simulink model "BLDCmotorControl_FOC_R2017b_fixdt"  (R2017b)
settings: Solver=FixedStepDiscrete  StartTime=0  StopTime=0.5  FixedStep=Ts  MaxStep=1e-6  RelTol=1e-6  AbsTol=1e-6  EnableMultiTasking=on
PreLoadFcn:
  | addpath(pwd);
  | addpath(genpath('01_Libraries'));
  | addpath(genpath('02_Figures'));
  | addpath(genpath('03_CreateParamTable'));
InitFcn:
  | init_model;
values from neighbouring files (symbols this model uses):
  a_elecAngle = 60    [init_model.m]
  a_elecPeriod = 360    [init_model.m]
  a_phaAdvMax = 25    [init_model.m]
  b_diagEna = 1    [init_model.m]
  b_fieldWeakEna = 0    [init_model.m]
  cf_currFilt = 0.12    [init_model.m]
  cf_idKi = 60 / (f_ctrl/3)    (= 0.01125)    [init_model.m]
  cf_idKp = 0.2    [init_model.m]
  cf_iqKi = 100 / (f_ctrl/3)    (= 0.01875)    [init_model.m]
  cf_iqKiLimProt = 60 / (f_ctrl/3)    (= 0.01125)    [init_model.m]
  cf_iqKp = 0.3    [init_model.m]
  cf_KbLimProt = 1000 / (f_ctrl/3)    (= 0.1875)    [init_model.m]
  cf_nKi = 20.4 / (f_ctrl/3)    (= 0.003825)    [init_model.m]
  cf_nKiLimProt = 20 / (f_ctrl/3)    (= 0.00375)    [init_model.m]
  cf_nKp = 1.18    [init_model.m]
  cf_speedCoef = round(f_ctrl * a_mechAngle * (pi/180) * (30/pi))    [init_model.m]
  CTRL_COM = 0    [init_model.m]
  CTRL_FOC = 2    [init_model.m]
  CTRL_SIN = 1    [init_model.m]
  dV_openRate = 1000 / (f_ctrl/3)    (= 0.1875)    [init_model.m]
  dz_cntTrnsDetHi = 40    [init_model.m]
  dz_cntTrnsDetLo = 20    [init_model.m]
  i_max = i_max * i_sca    (= 750)    [init_model.m]
  id_fieldWeakMax = 5 * i_sca    (= 250)    [init_model.m]
  iq_maxSca_M1 = sqrt(1 - iq_maxSca_XA.^2)    [init_model.m]
  n_commAcvLo = 15    [init_model.m]
  n_commDeacvHi = 30    [init_model.m]
  n_fieldWeakAuthHi = 400    [init_model.m]
  n_fieldWeakAuthLo = 300    [init_model.m]
  n_max = 1000    [init_model.m]
  n_polePairs = 15    [init_model.m]
  n_stdStillDet = 3    [init_model.m]
  OPEN_MODE = 0    [init_model.m]
  r_cos_M1 = cos((a_elecAngle_XA + 0)*(pi/180))    [init_model.m]
  r_errInpTgtThres = 600    [init_model.m]
  r_fieldWeakHi = 1500    [init_model.m]
  r_fieldWeakLo = 1000    [init_model.m]
  r_sin3PhaA_M1 = sin3Arm + A*r_sinPhaA_M1    [init_model.m]
  r_sin3PhaB_M1 = sin3Arm + A*r_sinPhaB_M1    [init_model.m]
  r_sin3PhaC_M1 = sin3Arm + A*r_sinPhaC_M1    [init_model.m]
  r_sin_M1 = sin((a_elecAngle_XA + 0)*(pi/180))    [init_model.m]
  SPD_MODE = 2    [init_model.m]
  t_errDequal = 1.80 * f_ctrl/3    (= 9600)    [init_model.m]
  t_errQual = 0.24 * f_ctrl/3    (= 1280)    [init_model.m]
  TRQ_MODE = 3    [init_model.m]
  Ts = 5e-6    (= 5e-06)    [init_model.m]
  Ts_ctrl = 6e-5    (= 6e-05)    [init_model.m]
  Vd_max = 1000 - V_margin    (= 900)    [init_model.m]
  vec_hallToPos = [0 2 0 1 4 3 5 0]    [init_model.m]
  VLT_MODE = 1    [init_model.m]
  Vq_max_M1 = sqrt(Vd_max^2 - Vq_max_XA.^2)    [init_model.m]
  z_commutMap_M1 = [-1 -1  0  1  1  0 ... (first row only)    [init_model.m]
  z_ctrlModReq = VLT_MODE    (= 1)    [init_model.m]
  z_ctrlTypSel = 2    [init_model.m]
  z_maxCntRst = 2000    [init_model.m]
  z_selPhaCurMeasABC = 0    [init_model.m]
undefined symbols (not defined in the file or in its folder): DiscIntNeverNeededParam, sigbuilder_block
libraries: BLDC_controller_Lib x15, simulink x14, powerlib x6, pePwmGenerator x1
(part 1 of 4)
Description:
  | This model implements FOC controller for a BLDC motor.
  | The controller is capable for embedded code generation.
  | 
  | Copyright © Emanuel FERU
settings Model: ExtModeAutoUpdateStatusClock=off  TunableVars=Vd_max,Vq_max_M1,Vq_max_XA,a_phaAdvMax,b_diagEna,b_fieldWeakEna,b_selPhaABCurrMeas,cf_KbLimProt,cf_currFilt,cf_idKi,cf_idKp,cf_iqKi,cf_iqKiLimProt,cf_iqKp,cf_nKi,cf_nKiLimProt,cf_nKp,cf_speedCoef,dV_openRate,dz_cntTrnsDetHi,dz_cntTrnsDetLo,i_max,id_fieldWeakMax,n_commAcvLo,n_commDeacvHi,n_fieldWeakAuthHi,n_fieldWeakAuthLo,n_max,n_stdStillDet,r_errInpTgtThres,r_fieldWeakHi,r_fieldWeakLo,t_errDequal,t_errQual,z_ctrlTypSel,z_maxCntRst,z_selPhaCurMeasABC  TunableVarsStorageClass=Auto,Auto,Auto,Auto,Auto,Auto,Auto,Auto,Auto,Auto,Auto,Auto,Auto,Auto,Auto,Auto,Auto,Auto,Auto,Auto,Auto,Auto,Auto,Auto,Auto,Auto,Auto,Auto,Auto,Auto,Auto,Auto,Auto,Auto,Auto,Auto,Auto  TunableVarsTypeQualifier=,,,,,,,,,,,,,,,,,,,,,,,,,,,,,,,,,,,,  Creator=MathWorks  LastModifiedBy=eferu
settings SolverCC: AutoInsertRateTranBlk=on
settings DataIOCC: LimitDataPoints=on  SaveFormat=Array  ReturnWorkspaceOutputs=on  SignalLoggingName=sigsOut
settings OptimizationCC: DefaultParameterBehavior=Inlined  UseDivisionForNetSlopeComputation=on  UseFloatMulNetSlope=on  UseSpecifiedMinMax=on  InlineInvariantSignals=on  PassReuseOutputArgsAs=Individual arguments  ExpressionDepthLimit=2147483647  ZeroExternalMemoryAtStartup=off  ZeroInternalMemoryAtStartup=off  NoFixptDivByZeroProtection=on  EfficientFloat2IntCast=on  LifeSpan=1  OptimizeBlockOrder=speed  DifferentSizesBufferReuse=on
settings DebuggingCC: ReadBeforeWriteMsg=DisableAll  WriteAfterWriteMsg=DisableAll  WriteAfterReadMsg=DisableAll  UnderspecifiedInitializationDetection=Classic  InheritedTsInSrcMsg=none  MultiTaskDSMMsg=none  MultiTaskCondExecSysMsg=none  ParameterTunabilityLossMsg=error  FcnCallInpInsideContextMsg=warning  UnconnectedInputMsg=error  UnconnectedOutputMsg=error  UnconnectedLineMsg=error  StateNameClashWarn=warning  SFUnexpectedBacktrackingDiag=warning  SFNoUnconditionalDefaultTransitionDiag=warning  SFExecutionAtInitializationDiag=none
settings HardwareCC: ProdBitPerPointer=32  ProdBitPerSizeT=32  ProdBitPerPtrDiffT=32  ProdLargestAtomicInteger=Long  ProdLargestAtomicFloat=Double  ProdWordSize=32  ProdHWDeviceType=ARM Compatible->ARM Cortex  TargetBitPerPointer=64  TargetBitPerSizeT=64  TargetBitPerPtrDiffT=64  TargetLongLongMode=on  TargetIntDivRoundTo=Zero  TargetEndianess=LittleEndian  TargetWordSize=64  TargetHWDeviceType=MATLAB Host  ProdEqTarget=off
settings ModelReferenceCC: UpdateModelReferenceTargets=IfOutOfDate  PropagateSignalLabelsOutOfModel=off
settings SFSimCC: SFSimEcho=off  MATLABDynamicMemAlloc=off
settings RTWCC: SystemTargetFile=ert.tlc  GenCodeOnly=on  TemplateMakefile=ert_default_tmf  GenerateReport=on  BuildConfiguration=Faster Runs  IncludeHyperlinkInReport=on  LaunchReport=on  GenerateTraceInfo=on  GenerateTraceReport=on  GenerateTraceReportSl=on  GenerateTraceReportSf=on  GenerateTraceReportEml=on  GenerateWebview=on  GenerateCodeMetricsReport=on  GenerateCodeReplacementReport=on
settings CodeAppCC: ForceParamTrailComments=on  IgnoreCustomStorageClasses=off  OperatorAnnotations=on  SimulinkDataObjDesc=on  SFDataObjDesc=on  CustomSymbolStrGlobalVar=rt$N$M  CustomSymbolStrType=$N$M  CustomSymbolStrFcn=$N$M$F  CustomSymbolStrMacro=$N$M  InsertBlockDesc=on
settings ERTTargetCC: GenerateSampleERTMain=on  IncludeMdlTerminateFcn=off  CombineSignalStateStructs=on  SuppressErrorStatus=on  MultiInstanceERTCode=on  CodeInterfacePackaging=Reusable function  SupportNonFinite=off  SupportComplex=off  InlinedParameterPlacement=NonHierarchical  RootIOFormat=Part of model data structure  ERTCustomFileTemplate=example_file_process.tlc  ERTFilePackagingFormat=CompactWithDataFile  PreserveStaticInFcnDecls=off
settings ConfigComp: CovMetricSettings=dw  CovHtmlReporting=on  CovSaveCumulativeToWorkspaceVar=on  CovSaveSingleToWorkspaceVar=on  CovExternalEMLEnable=off  CovSFcnEnable=off
settings SimscapeCC: SimscapeNormalizeSystem=off

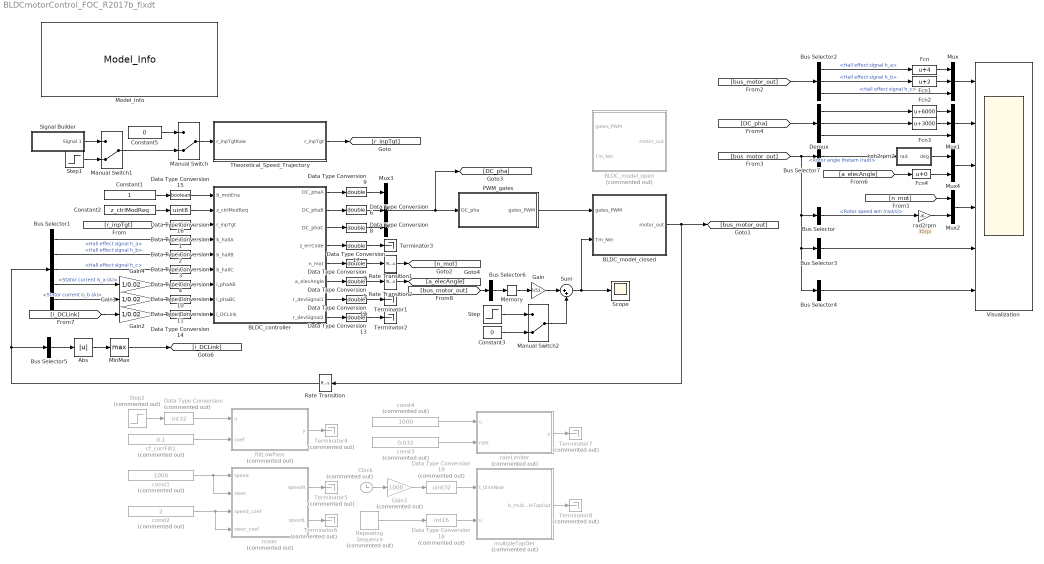
== system BLDCmotorControl_FOC_R2017b_fixdt ==
  Abs : Abs
  BLDC_controller : Subsystem  TreatAsAtomicUnit=on  SystemSampleTime=Ts_ctrl
  BLDC_model_closed : Subsystem
      mask help: Simulink:masks:GenSFuncDesc_MD
      mask Help: eval('feval(''rtwprivate'',''rtwhelpview'',''rtw_sfcn_block'')');
  BLDC_model_open : Subsystem  Commented=on
  Bus Selector : BusSelector  OutputSignals=Rotor speed wm (rad/s)
  Bus Selector1 : BusSelector  OutputSignals=Hall effect signal h_a,Hall effect signal h_b,Hall effect signal h_c,Stator current is_a (A),Stator current is_b (A)
  Bus Selector2 : BusSelector  OutputSignals=Hall effect signal h_a,Hall effect signal h_b,Hall effect signal h_c
  Bus Selector3 : BusSelector  OutputSignals=Stator current is_a (A),Stator current is_b (A),Stator current is_c (A),Electromagnetic torque Te (N*m)  OutputAsBus=on
  Bus Selector4 : BusSelector  OutputSignals=Stator back EMF e_a (V),Stator back EMF e_b (V),Stator back EMF e_cV)  OutputAsBus=on
  Bus Selector5 : BusSelector  OutputSignals=Stator current is_a (A),Stator current is_b (A),Stator current is_c (A)  OutputAsBus=on
  Bus Selector6 : BusSelector  OutputSignals=Rotor speed wm (rad/s)  OutputAsBus=on
  Bus Selector7 : BusSelector  OutputSignals=Rotor angle thetam (rad)
  Clock : Clock  Commented=on
  Constant1 : Constant  OutDataTypeStr=double
  Constant2 : Constant  Value=z_ctrlModReq  OutDataTypeStr=double
  Constant3 : Constant  Value=0  OutDataTypeStr=double
  Constant5 : Constant  Value=0  OutDataTypeStr=double
  Data Type Conversion : DataTypeConversion  Commented=on  OutDataTypeStr=int32
  Data Type Conversion{1,10..11,14} (4 alike) : DataTypeConversion  OutDataTypeStr=int16  RndMeth=Zero
  Data Type Conversion{5..9,12..13,17} (8 alike) : DataTypeConversion  OutDataTypeStr=double  RndMeth=Zero
  Data Type Conversion15 : DataTypeConversion  OutDataTypeStr=boolean  RndMeth=Zero
  Data Type Conversion{2..4,16} (4 alike) : DataTypeConversion  OutDataTypeStr=uint8  RndMeth=Zero
  Data Type Conversion18 : DataTypeConversion  Commented=on  OutDataTypeStr=int16
  Data Type Conversion19 : DataTypeConversion  Commented=on  OutDataTypeStr=uint32
  Demux : Demux  Outputs=3
  Fcn : Fcn  Expr=u+4
  Fcn1 : Fcn  Expr=u+2
  Fcn2 : Fcn  Expr=u+6000
  Fcn3 : Fcn  Expr=u+3000
  Fcn4 : Fcn  Expr=u+0
  Gain : Gain  Gain=5/52
  Gain1 : Gain  Tag=struct('comment',struct('text','','placement',1),'logdata',struct('maxnumvals',inf,'plotchannels',[],'loggingmode',3,'channels',1),'output',struct('variable','','description','','name','$S_$B','width',1,'address','','max',NaN,'min',NaN,'class','default','type','CONTINUOUS','scaling','','lsb',1,'offset',0,'arb',0,'freeze',1,'unit','','autoscalingmode',1,'lowerheadroom',1,'upperheadroom',1,'headroomunit','bit','keepdatatype',1,'checkmin',0,'checkmax',0,'castoutput',0,'show',0),'gain',struct('variable','','description','','name','$S_$B_gain','width',1,'address','','max',NaN,'min',NaN,'class','default','type','CONTINUOUS','scaling','','lsb',1,'offset',0,'arb',0,'freeze',1,'unit','','keepdatatype',1,'value','1','scalar',0,'tolerance',1),'scalingvalid',0,'date',730486)  Gain=1/0.02  RndMeth=Zero  SaturateOnIntegerOverflow=on  OutDataTypeStr=Inherit: Same as input  ParamDataTypeStr=Inherit: Same as input
  Gain2 : Gain  Tag=struct('comment',struct('text','','placement',1),'logdata',struct('maxnumvals',inf,'plotchannels',[],'loggingmode',3,'channels',1),'output',struct('variable','','description','','name','$S_$B','width',1,'address','','max',NaN,'min',NaN,'class','default','type','CONTINUOUS','scaling','','lsb',1,'offset',0,'arb',0,'freeze',1,'unit','','autoscalingmode',1,'lowerheadroom',1,'upperheadroom',1,'headroomunit','bit','keepdatatype',1,'checkmin',0,'checkmax',0,'castoutput',0,'show',0),'gain',struct('variable','','description','','name','$S_$B_gain','width',1,'address','','max',NaN,'min',NaN,'class','default','type','CONTINUOUS','scaling','','lsb',1,'offset',0,'arb',0,'freeze',1,'unit','','keepdatatype',1,'value','1','scalar',0,'tolerance',1),'scalingvalid',0,'date',730486)  Gain=1/0.02  RndMeth=Zero  SaturateOnIntegerOverflow=on  OutDataTypeStr=Inherit: Same as input  ParamDataTypeStr=Inherit: Same as input
  Gain3 : Gain  Tag=struct('comment',struct('text','','placement',1),'logdata',struct('maxnumvals',inf,'plotchannels',[],'loggingmode',3,'channels',1),'output',struct('variable','','description','','name','$S_$B','width',1,'address','','max',NaN,'min',NaN,'class','default','type','CONTINUOUS','scaling','','lsb',1,'offset',0,'arb',0,'freeze',1,'unit','','autoscalingmode',1,'lowerheadroom',1,'upperheadroom',1,'headroomunit','bit','keepdatatype',1,'checkmin',0,'checkmax',0,'castoutput',0,'show',0),'gain',struct('variable','','description','','name','$S_$B_gain','width',1,'address','','max',NaN,'min',NaN,'class','default','type','CONTINUOUS','scaling','','lsb',1,'offset',0,'arb',0,'freeze',1,'unit','','keepdatatype',1,'value','1','scalar',0,'tolerance',1),'scalingvalid',0,'date',730486)  Commented=on  Gain=1000  RndMeth=Zero  SaturateOnIntegerOverflow=on  OutDataTypeStr=Inherit: Same as input  ParamDataTypeStr=Inherit: Same as input
  Gain4 : Gain  Tag=struct('comment',struct('text','','placement',1),'logdata',struct('maxnumvals',inf,'plotchannels',[],'loggingmode',3,'channels',1),'output',struct('variable','','description','','name','$S_$B','width',1,'address','','max',NaN,'min',NaN,'class','default','type','CONTINUOUS','scaling','','lsb',1,'offset',0,'arb',0,'freeze',1,'unit','','autoscalingmode',1,'lowerheadroom',1,'upperheadroom',1,'headroomunit','bit','keepdatatype',1,'checkmin',0,'checkmax',0,'castoutput',0,'show',0),'gain',struct('variable','','description','','name','$S_$B_gain','width',1,'address','','max',NaN,'min',NaN,'class','default','type','CONTINUOUS','scaling','','lsb',1,'offset',0,'arb',0,'freeze',1,'unit','','keepdatatype',1,'value','1','scalar',0,'tolerance',1),'scalingvalid',0,'date',730486)  Gain=1/0.02  RndMeth=Zero  SaturateOnIntegerOverflow=on  OutDataTypeStr=Inherit: Same as input  ParamDataTypeStr=Inherit: Same as input
  Manual Switch : ManualSwitch  CurrentSetting=0
  Manual Switch1 : ManualSwitch  CurrentSetting=0
  Manual Switch2 : ManualSwitch  CurrentSetting=0
  Memory : Memory
  MinMax : MinMax  Function=max
  Model_Info : BLDC_controller_Lib/Model_Info
  Mux : Mux  Inputs=3
  Mux1 : Mux  Inputs=3
  Mux2 : Mux  Inputs=2
  Mux3 : Mux  Inputs=3
  Mux4 : Mux  Inputs=2
  PWM_gates : Subsystem
  Rate Transition : RateTransition  Integrity=off  Deterministic=off
  Rate Transition1 : RateTransition
  Rate Transition2 : RateTransition
  Repeating Sequence : simulink/Sources/Repeating Sequence  Commented=on  rep_seq_t=[0 0.4 0.8 1.2 1.6 3]  rep_seq_y="[0 900  0  900 0 0]"
  Scope : Scope
  Signal Builder : Subsystem  Tag=STV Subsys  LoadFcn=sigbuilder_block('load');  StartFcn=sigbuilder_block('start');  StopFcn=sigbuilder_block('stop');  ClipboardFcn=sigbuilder_block('clipboard');  mask(Sigbuilder block){tuvar=[0:10]}
      mask help: Simulink:masks:SigbuilderBlock_MD
      mask init:
      | if ~strcmp(get_param(bdroot(gcbh),'SimulationStatus'),'stopped') tuvar = sigbuilder_block('maskInit'); end
      settings: CopyFcn=sigbuilder_block('copy');  DeleteFcn=sigbuilder_block('delete');  ModelCloseFcn=sigbuilder_block('modelClose');  PreSaveFcn=sigbuilder_block('preSave');  PauseFcn=sigbuilder_block('pause');  ContinueFcn=sigbuilder_block('continue');  NameChangeFcn=sigbuilder_block('namechange');  OpenFcn=sigbuilder_block('open',[141.283 165.057 550.868 400.075 ]);  CloseFcn=sigbuilder_block('close');
      mask Display: plot(0, 0, 100, 100,[2, 2, 32, 32, 2], [68, 8, 8, 68, 68],[32, 2], [38, 38], [32, 19, 2],[53, 60, 44], [32, 17, 17, 2],[16, 16, 31, 31]);txt = getActiveGroup(gcbh);text(2, 100, txt,'verticalAlignment', 'top');
  Step : Step  Time=0.25  Before=-5  After=5  SampleTime=0
  Step1 : Step  Time=0.25  Before=1500  After=-1500
  Step2 : Step  Commented=on  Time=0.25  Before=20000  After=0  SampleTime=0
  Sum : Sum  Inputs=|++
  Terminator1 : Terminator
      settings: Tag=Controls_Lib  Description=Terminator  CopyFcn=Lib_CopyFcn(gcb);  PreDeleteFcn=Lib_PreDeleteFcn(gcb);
  Terminator2 : Terminator
      settings: Tag=Controls_Lib  Description=Terminator  CopyFcn=Lib_CopyFcn(gcb);  PreDeleteFcn=Lib_PreDeleteFcn(gcb);
  Terminator3 : Terminator
      settings: Tag=Controls_Lib  Description=Terminator  CopyFcn=Lib_CopyFcn(gcb);  PreDeleteFcn=Lib_PreDeleteFcn(gcb);
  Terminator{4..8} (5 alike) : Terminator  Commented=on
      settings: Tag=Controls_Lib  Description=Terminator  CopyFcn=Lib_CopyFcn(gcb);  PreDeleteFcn=Lib_PreDeleteFcn(gcb);
  Theoretical_Speed_Trajectory : Subsystem
  Visualization : Scope  NumInputPorts=6
  cf_currFilt1 : Constant  Commented=on  Value=0.1  OutDataTypeStr=fixdt(0,16,16)
  const1 : Constant  Commented=on  Value=1000  OutDataTypeStr=fixdt(1,16,4)
  const2 : Constant  Commented=on  Value=2  OutDataTypeStr=fixdt(1,16,14)
  const3 : Constant  Commented=on  Value=0.032  OutDataTypeStr=fixdt(1,16,4)
  const4 : Constant  Commented=on  Value=1000  OutDataTypeStr=int16
  filtLowPass : Subsystem  Commented=on  TreatAsAtomicUnit=on  SystemSampleTime=Ts_ctrl
      settings: RTWFcnNameOpts=Use subsystem name
  kph2rpm2 : Subsystem
  mixer : Subsystem  Commented=on  TreatAsAtomicUnit=on  SystemSampleTime=Ts_ctrl
      settings: RTWFcnNameOpts=Use subsystem name
  multipleTapDet : Subsystem  Commented=on  TreatAsAtomicUnit=on
      settings: RTWFcnNameOpts=Use subsystem name
  rad2rpm : Gain  Gain=30/pi
  rateLimiter : Subsystem  Commented=on  TreatAsAtomicUnit=on  SystemSampleTime=Ts_ctrl
      settings: RTWFcnNameOpts=Use subsystem name
  wires:
  Mux2/1 -> Visualization/4
  Bus Selector/1 -> rad2rpm/1  "<Rotor speed wm (rad/s)>"
  Bus Selector2/3 -> Mux/3  "<Hall effect signal h_c>"
  Bus Selector2/2 -> Fcn1/1  "<Hall effect signal h_b>"
  Bus Selector2/1 -> Fcn/1  "<Hall effect signal h_a>"
  Fcn1/1 -> Mux/2
  Mux/1 -> Visualization/1
  Fcn/1 -> Mux/1
  Demux/1 -> Fcn2/1
  Demux/2 -> Fcn3/1
  Fcn2/1 -> Mux1/1
  Fcn3/1 -> Mux1/2
  Demux/3 -> Mux1/3
  Mux1/1 -> Visualization/2
  Bus Selector4/1 -> Visualization/6
  rad2rpm/1 -> Mux2/2
  BLDC_controller/5(n_mot) -> Data Type Conversion7/1
  Sum/1 -> BLDC_model_closed/2(Tm_Nm), Scope/1
  Bus Selector1/2 -> Data Type Conversion3/1  "<Hall effect signal h_b>"
  Bus Selector1/1 -> Data Type Conversion2/1  "<Hall effect signal h_a>"
  Bus Selector1/3 -> Data Type Conversion4/1  "<Hall effect signal h_c>"
  Data Type Conversion2/1 -> BLDC_controller/4("b_hallA ")
  Data Type Conversion3/1 -> BLDC_controller/5(b_hallB)
  Data Type Conversion4/1 -> BLDC_controller/6(b_hallC)
  Theoretical_Speed_Trajectory/1(r_inpTgt) -> [r_inpTgt]
  [r_inpTgt] -> Data Type Conversion1/1
  Data Type Conversion1/1 -> BLDC_controller/3(r_inpTgt)
  BLDC_controller/2(DC_phaB) -> Data Type Conversion6/1
  BLDC_controller/3(DC_phaC) -> Data Type Conversion8/1
  BLDC_controller/1(DC_phaA) -> Data Type Conversion9/1
  BLDC_controller/6(a_elecAngle) -> Data Type Conversion5/1
  Mux3/1 -> [DC_pha], PWM_gates/1(DC_pha)
  PWM_gates/1(gates_PWM) -> BLDC_model_closed/1(gates_PWM)
  Data Type Conversion7/1 -> Rate Transition1/1
  [n_mot] -> Mux2/1
  [bus_motor_out] -> Bus Selector2/1
  [bus_motor_out] -> Bus Selector7/1, Bus Selector3/1, Bus Selector4/1, Bus Selector/1
  [DC_pha] -> Demux/1
  Manual Switch/1 -> Theoretical_Speed_Trajectory/1(r_inpTgtRaw)
  Constant5/1 -> Manual Switch/1
  Signal Builder/1(Signal 1) -> Manual Switch1/1
  Manual Switch1/1 -> Manual Switch/2
  Step1/1 -> Manual Switch1/2
  Data Type Conversion5/1 -> Rate Transition2/1
  Data Type Conversion8/1 -> Mux3/3
  Data Type Conversion6/1 -> Mux3/2
  Data Type Conversion9/1 -> Mux3/1
  Data Type Conversion10/1 -> BLDC_controller/7(i_phaAB)
  Data Type Conversion11/1 -> BLDC_controller/8(i_phaBC)
  Gain4/1 -> Data Type Conversion10/1
  Gain1/1 -> Data Type Conversion11/1
  BLDC_controller/7(r_devSignal1) -> Data Type Conversion12/1
  Data Type Conversion13/1 -> Terminator2/1
  BLDC_controller/8(r_devSignal2) -> Data Type Conversion13/1
  Gain2/1 -> Data Type Conversion14/1
  Data Type Conversion14/1 -> BLDC_controller/9(i_DCLink)
  [i_DCLink] -> Gain2/1
  Bus Selector1/4 -> Gain4/1  "<Stator current is_a (A)>"
  Bus Selector1/5 -> Gain1/1  "<Stator current is_b (A)>"
  Data Type Conversion15/1 -> BLDC_controller/1(b_motEna)
  Constant1/1 -> Data Type Conversion15/1
  [bus_motor_out] -> Bus Selector6/1
  Bus Selector6/1 -> Memory/1
  Gain/1 -> Sum/1
  Data Type Conversion16/1 -> BLDC_controller/2(z_ctrlModReq)
  Constant2/1 -> Data Type Conversion16/1
  Rate Transition/1 -> Bus Selector1/1, Bus Selector5/1
  Memory/1 -> Gain/1
  Step/1 -> Manual Switch2/1
  Manual Switch2/1 -> Sum/2
  Constant3/1 -> Manual Switch2/2
  Data Type Conversion17/1 -> Terminator3/1
  BLDC_controller/4(z_errCode) -> Data Type Conversion17/1
  Data Type Conversion12/1 -> Terminator1/1
  Bus Selector5/1 -> Abs/1
  BLDC_model_closed/1(motor_out) -> Rate Transition/1, [bus_motor_out]
  MinMax/1 -> [i_DCLink]
  Abs/1 -> MinMax/1
  filtLowPass/1(y) -> Terminator4/1
  cf_currFilt1/1 -> filtLowPass/2(coef)
  Data Type Conversion/1 -> filtLowPass/1(u)
  mixer/1(speedR) -> Terminator5/1
  const1/1 -> mixer/2(steer), mixer/1(speed)
  const2/1 -> mixer/4(steer_coef), mixer/3(speed_coef)
  mixer/2(speedL) -> Terminator6/1
  const3/1 -> rateLimiter/2(rate)
  const4/1 -> rateLimiter/1(u)
  rateLimiter/1(y) -> Terminator7/1
  Gain3/1 -> Data Type Conversion19/1
  Data Type Conversion19/1 -> multipleTapDet/1(t_timeNow)
  Data Type Conversion18/1 -> multipleTapDet/2(u)
  multipleTapDet/1(b_multipleTapOut) -> Terminator8/1
  Repeating Sequence/1 -> Data Type Conversion18/1
  Clock/1 -> Gain3/1
  Step2/1 -> Data Type Conversion/1
  Bus Selector7/1 -> kph2rpm2/1(rad)  "<Rotor angle thetam (rad)>"
  Rate Transition1/1 -> [n_mot]
  Rate Transition2/1 -> [a_elecAngle]
  Bus Selector3/1 -> Visualization/5
  Mux4/1 -> Visualization/3
  [a_elecAngle] -> Fcn4/1
  kph2rpm2/1(deg) -> Mux4/1
  Fcn4/1 -> Mux4/2

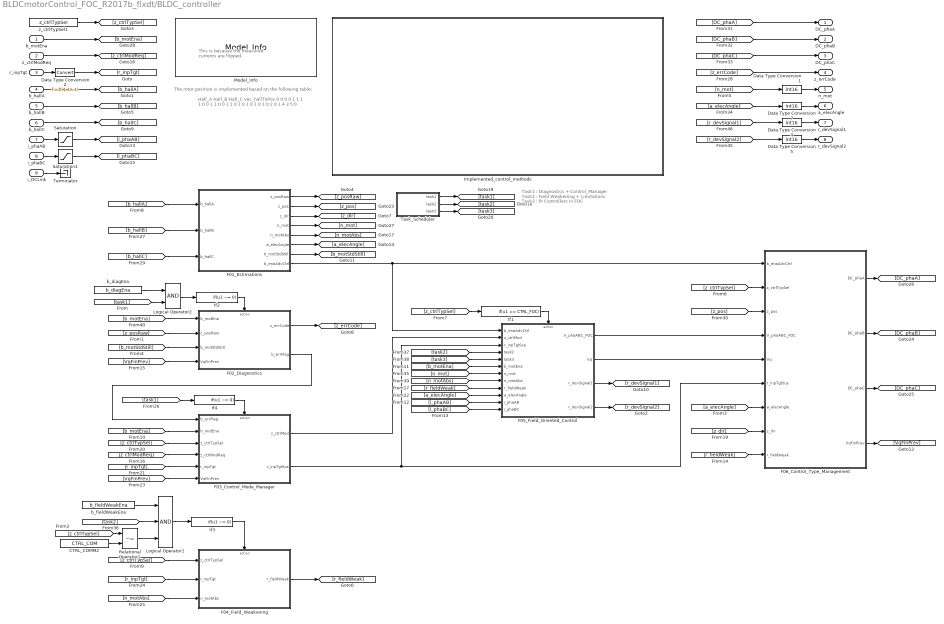
== system BLDCmotorControl_FOC_R2017b_fixdt/BLDC_controller ==
  note: Task1 : Diagnostics + Control_Manager
      | Task2 : Field Weakening + Limitations
      | Task3 : PI Controllers in FOC
  note: The rotor position is implemented based on the following table:
  note: Hall_A
      | Hall_B
      | Hall_C
      | vec_hallToPos
      |
      | 0
      | 0
      | 0
      | 0
      | 1
      | 1
      | 1
      | 1
      | 0
      | 0
      | 1
      | 1
      | 0
      | 0
      | 1
      | 1
      | 0
      | 1
      | 0
      | 1
      | 0
      | 1
      | 0
      | 1
      | 0
      | 2
      | 0
      | 1
      | 4
      | 3
      | 5
      | 0
  note: This is because the measured currents are flipped.
  b_motEna : Inport
  z_ctrlModReq : Inport  Port=2
  r_inpTgt : Inport  Port=3
  "b_hallA " : Inport  Port=4
  b_hallB : Inport  Port=5
  b_hallC : Inport  Port=6
  i_phaAB : Inport  Port=7
  i_phaBC : Inport  Port=8
  i_DCLink : Inport  Port=9
  CTRL_COMM2 : Constant  Value=CTRL_COM  OutDataTypeStr=Inherit: Inherit via back propagation
  Data Type Conversion{1,4..5,7} (4 alike) : DataTypeConversion  OutDataTypeStr=int16
  Data Type Conversion2 : DataTypeConversion  OutDataTypeStr=fixdt(1,16,4)  SaturateOnIntegerOverflow=on
  F01_Estimations : Subsystem
  F02_Diagnostics : Subsystem
  F03_Control_Mode_Manager : Subsystem
  F04_Field_Weakening : Subsystem
  F05_Field_Oriented_Control : Subsystem
  F06_Control_Type_Management : Subsystem
  If1 : If  IfExpression=u1 == CTRL_FOC  ShowElse=off
  If2 : If  IfExpression=u1 ~= 0  ShowElse=off
  If3 : If  IfExpression=u1 ~= 0  ShowElse=off
  If4 : If  IfExpression=u1 ~= 0  ShowElse=off
  Implemented_control_methods : Subsystem
      mask Display: image('control_methods.png')
  Logical Operator1 : Logic  Inputs=3  AllPortsSameDT=off  OutDataTypeStr=boolean
  Logical Operator2 : Logic  AllPortsSameDT=off  OutDataTypeStr=boolean
  Model_Info : BLDC_controller_Lib/Model_Info
  Relational Operator1 : RelationalOperator  Operator=~=  OutDataTypeStr=boolean  RndMeth=Simplest
  Saturation : Saturate  UpperLimit=1700  LowerLimit=-1700  OutDataTypeStr=fixdt(1,16,4)
  Saturation1 : Saturate  UpperLimit=1700  LowerLimit=-1700  OutDataTypeStr=fixdt(1,16,4)
  Task_Scheduler : Subsystem
  Terminator : Terminator
  b_diagEna : Constant  Value=b_diagEna  OutDataTypeStr=boolean
  b_fieldWeakEna : Constant  Value=b_fieldWeakEna  OutDataTypeStr=boolean
  z_ctrlTypSel1 : Constant  Value=z_ctrlTypSel  OutDataTypeStr=uint8
  DC_phaA : Outport
  DC_phaB : Outport  Port=2
  DC_phaC : Outport  Port=3
  z_errCode : Outport  Port=4  OutputWhenDisabled=reset  InitialOutput=0
  n_mot : Outport  Port=5
  a_elecAngle : Outport  Port=6
  r_devSignal1 : Outport  Port=7  OutputWhenDisabled=reset  InitialOutput=0
  r_devSignal2 : Outport  Port=8  OutputWhenDisabled=reset  InitialOutput=0
  wires:
  [n_mot] -> F05_Field_Oriented_Control/7(n_mot)
  F02_Diagnostics/2(b_errFlag) -> F03_Control_Mode_Manager/1(b_errFlag)
  Data Type Conversion5/1 -> r_devSignal2/1
  Data Type Conversion4/1 -> r_devSignal1/1
  If1/1 -> F05_Field_Oriented_Control/Action
  i_phaBC/1 -> Saturation1/1
  [r_devSignal1] -> Data Type Conversion4/1
  [z_ctrlTypSel] -> If1/1
  [z_pos] -> F06_Control_Type_Management/3(z_pos)
  Saturation/1 -> [i_phaAB]
  F01_Estimations/5(n_motAbs) -> [n_motAbs]
  [b_motEna] -> F03_Control_Mode_Manager/2(b_motEna)
  [z_errCode] -> z_errCode/1
  If2/1 -> F02_Diagnostics/Action
  [r_fieldWeak] -> F05_Field_Oriented_Control/9(r_fieldWeak)
  [DC_phaB] -> DC_phaB/1
  [z_ctrlTypSel] -> F06_Control_Type_Management/2(z_ctrlTypSel)
  [z_ctrlModReq] -> F03_Control_Mode_Manager/4(z_ctrlModReq)
  [z_posRaw] -> F02_Diagnostics/2(z_posRaw)
  Data Type Conversion1/1 -> n_mot/1
  Data Type Conversion2/1 -> [r_inpTgt]
  [i_phaAB] -> F05_Field_Oriented_Control/11(i_phaAB)
  i_phaAB/1 -> Saturation/1
  F05_Field_Oriented_Control/1(V_phaABC_FOC) -> F06_Control_Type_Management/4(V_phaABC_FOC)
  [i_phaBC] -> F05_Field_Oriented_Control/12(i_phaBC)
  [n_mot] -> Data Type Conversion1/1
  [a_elecAngle] -> Data Type Conversion7/1
  [DC_phaC] -> DC_phaC/1
  F06_Control_Type_Management/2(DC_phaB) -> [DC_phaB]
  z_ctrlModReq/1 -> [z_ctrlModReq]
  F06_Control_Type_Management/1(DC_phaA) -> [DC_phaA]
  F01_Estimations/4("n_mot ") -> [n_mot]
  F05_Field_Oriented_Control/4(r_devSignal2) -> [r_devSignal2]
  F01_Estimations/6(a_elecAngle) -> [a_elecAngle]
  [b_hallB] -> F01_Estimations/2(b_hallB)
  i_DCLink/1 -> Terminator/1
  F05_Field_Oriented_Control/3(r_devSignal1) -> [r_devSignal1]
  Data Type Conversion7/1 -> a_elecAngle/1
  F06_Control_Type_Management/3("DC_phaC ") -> [DC_phaC]
  Saturation1/1 -> [i_phaBC]
  b_hallB/1 -> [b_hallB]
  F01_Estimations/8(b_enaAdvCtrl) -> F05_Field_Oriented_Control/1(b_enaAdvCtrl), F06_Control_Type_Management/1(b_enaAdvCtrl)
  F02_Diagnostics/1("z_errCode ") -> [z_errCode]
  b_motEna/1 -> [b_motEna]
  b_hallC/1 -> [b_hallC]
  [a_elecAngle] -> F05_Field_Oriented_Control/10(a_elecAngle)
  [DC_phaA] -> DC_phaA/1
  F01_Estimations/1(z_posRaw) -> [z_posRaw]
  r_inpTgt/1 -> Data Type Conversion2/1
  F03_Control_Mode_Manager/1(z_ctrlMod) -> F05_Field_Oriented_Control/2(z_ctrlMod)
  [b_hallA] -> F01_Estimations/1(b_hallA)
  [r_devSignal2] -> Data Type Conversion5/1
  "b_hallA "/1 -> [b_hallA]
  F01_Estimations/2(z_pos) -> [z_pos]
  z_ctrlTypSel1/1 -> [z_ctrlTypSel]
  [b_hallC] -> F01_Estimations/3(b_hallC)
  [b_motStdStill] -> F02_Diagnostics/3(b_motStdStill)
  F01_Estimations/7(b_motStdStill) -> [b_motStdStill]
  [VqFinPrev] -> F02_Diagnostics/4(VqFinPrev)
  F06_Control_Type_Management/4(VqFinPrev) -> [VqFinPrev]
  [b_motEna] -> F05_Field_Oriented_Control/6(b_motEna)
  F03_Control_Mode_Manager/2(r_inpTgtSca) -> F05_Field_Oriented_Control/3(r_inpTgtSca), F06_Control_Type_Management/6(r_inpTgtSca)
  F05_Field_Oriented_Control/2(Vq) -> F06_Control_Type_Management/5(Vq)
  [a_elecAngle] -> F06_Control_Type_Management/7(a_elecAngle)
  [r_fieldWeak] -> F06_Control_Type_Management/9(r_fieldWeak)
  F01_Estimations/3(z_dir) -> [z_dir]
  [z_dir] -> F06_Control_Type_Management/8(z_dir)
  [z_ctrlTypSel] -> F03_Control_Mode_Manager/3(z_ctrlTypSel)
  [r_inpTgt] -> F03_Control_Mode_Manager/5(r_inpTgt)
  [VqFinPrev] -> F03_Control_Mode_Manager/6(VqFinPrev)
  Logical Operator1/1 -> If3/1
  [z_ctrlTypSel] -> Relational Operator1/1
  CTRL_COMM2/1 -> Relational Operator1/2
  Relational Operator1/1 -> Logical Operator1/3
  b_fieldWeakEna/1 -> Logical Operator1/1
  F04_Field_Weakening/1("r_fieldWeak ") -> [r_fieldWeak]
  [z_ctrlTypSel] -> F04_Field_Weakening/1(z_ctrlTypSel)
  [r_inpTgt] -> F04_Field_Weakening/2(r_inpTgt)
  [n_motAbs] -> F04_Field_Weakening/3(n_motAbs)
  Task_Scheduler/3(task3) -> [task3]
  Task_Scheduler/2(task2) -> [task2]
  Task_Scheduler/1(task1) -> [task1]
  b_diagEna/1 -> Logical Operator2/1
  [task1] -> Logical Operator2/2
  Logical Operator2/1 -> If2/1
  If4/1 -> F03_Control_Mode_Manager/Action
  [task1] -> If4/1
  [task3] -> F05_Field_Oriented_Control/5(task3)
  [task2] -> F05_Field_Oriented_Control/4(task2)
  If3/1 -> F04_Field_Weakening/Action
  [task2] -> Logical Operator1/2
  [n_motAbs] -> F05_Field_Oriented_Control/8(n_motAbs)
  [b_motEna] -> F02_Diagnostics/1(b_motEna)

== system BLDCmotorControl_FOC_R2017b_fixdt/BLDC_model_closed ==
  gates_PWM : Inport
  Tm_Nm : Inport  Port=2
  BLDC_model_sfcn : S-Function  FunctionName=BLDC_model_sf  SFunctionModules=""  SFunctionDeploymentMode=off  EnableBusSupport=off  SFcnStateName=DWORK0  mask{rtw_sf_name=BLDC_model_sf, showVar=off}
      mask prompts: rtw_sf_name "Simulink:masks:GenSFuncName_MP"; showVar "Simulink:masks:GenSFuncShowModuleList_MP"
      mask help: Simulink:masks:GenSFuncDesc_MD
      mask init:
      | displist = '';
      | if ~strcmp(get_param(gcb, 'FunctionName'), rtw_sf_name);
      |   set_param(gcb, 'FunctionName', rtw_sf_name);
      | end
      | % Check if we are generating code
      | rtw_mode = false;
      | if strcmpi(get_param(bdroot(gcb),'SimulationStatus'),'Initializing')
      | 	rtw_mode = strcmpi(get_param(bdroot(gcb),'BuildingRTWCode'),'on') && ...
      | 		~strcmpi(get_param(bdroot(gcb),'TargetStyle'),'SimulationTarget');
      | end
      | if showVar || rtw_mode
      | 	if exist('rtwsfunc') == 2 | exist('rtwsfunc') == 6
      | 		tmplist = rtwsfunc(rtw_sf_name,gcb);
      | 		tmplist = DAStudio.message('Simulink:masks:GenSFuncListOfModules_IC', tmplist);
      | 	elseif showVar
      | 		tmplist1 = DAStudio.message('Simulink:masks:GenSFuncListOfModules_IC', '');
      |         tmplist2 = DAStudio.message('Simulink:masks:GenSFuncNotLicensed_IC');
      |         tmplist = [tmplist1 tmplist2];
      |  	end
      | end
      | if showVar
      |   displist = tmplist;
      | end
      settings: SFcnIsStateOwnerBlock=on
      settings: CopyFcn=|
      | if ~strcmp(get_param(gcb,'Linkstatus'),'none') && ...
      | ~strcmp(get_param(gcb,'Linkstatus'),'implicit')
      |   set_param(gcb,'LinkStatus','none');
      | end
      mask Help: eval('feval(''rtwprivate'',''rtwhelpview'',''rtw_sfcn_block'')');
      mask Display:
      | port_label('input',1,'gates_PWM');
      | port_label('input',2,'Tm_Nm');
      | port_label('output',1,'Stator current is_a (A)');
      | port_label('output',2,'Stator current is_b (A)');
      | port_label('output',3,'Stator current is_c (A)');
      | port_label('output',4,'Stator back EMF e_a (V)');
      | port_label('output',5,'Stator back EMF e_b (V)');
      | port_label('output',6,'Stator back EMF e_cV)');
      | port_label('output',7,'Hall effect signal h_a');
      | port_label('output',8,'Hall effect signal h_b');
      | port_label('output',9,'Hall effect signal h_c');
      | port_label('output',10,'Rotor speed wm (rad/s)');
      | port_label('output',11,'Rotor angle thetam (rad)');
      | port_label('output',12,'Electromagnetic torque Te (N*m)');
  __InputSSForSFun__ : Subsystem
  __OutputSSForSFun__ : Subsystem
  motor_out : Outport
  wires:
  gates_PWM/1 -> __InputSSForSFun__/1(gates_PWM)
  Tm_Nm/1 -> __InputSSForSFun__/2(Tm_Nm)
  __InputSSForSFun__/1(__UniqueOutportName__1__) -> BLDC_model_sfcn/1
  __InputSSForSFun__/2(__UniqueOutportName__2__) -> BLDC_model_sfcn/2
  BLDC_model_sfcn/1 -> __OutputSSForSFun__/1(__UniqueInportName__1__)
  BLDC_model_sfcn/2 -> __OutputSSForSFun__/2(__UniqueInportName__2__)
  BLDC_model_sfcn/3 -> __OutputSSForSFun__/3(__UniqueInportName__3__)
  BLDC_model_sfcn/4 -> __OutputSSForSFun__/4(__UniqueInportName__4__)
  BLDC_model_sfcn/5 -> __OutputSSForSFun__/5(__UniqueInportName__5__)
  BLDC_model_sfcn/6 -> __OutputSSForSFun__/6(__UniqueInportName__6__)
  BLDC_model_sfcn/7 -> __OutputSSForSFun__/7(__UniqueInportName__7__)
  BLDC_model_sfcn/8 -> __OutputSSForSFun__/8(__UniqueInportName__8__)
  BLDC_model_sfcn/9 -> __OutputSSForSFun__/9(__UniqueInportName__9__)
  BLDC_model_sfcn/10 -> __OutputSSForSFun__/10(__UniqueInportName__10__)
  BLDC_model_sfcn/11 -> __OutputSSForSFun__/11(__UniqueInportName__11__)
  BLDC_model_sfcn/12 -> __OutputSSForSFun__/12(__UniqueInportName__12__)
  __OutputSSForSFun__/1(motor_out) -> motor_out/1

== system BLDCmotorControl_FOC_R2017b_fixdt/BLDC_model_open ==
  gates_PWM : Inport
  Tm_Nm : Inport  Port=2
  Constant1 : Constant  Value=36
  Controlled Voltage Source1 : powerlib/Electrical Sources/Controlled Voltage Source  Initialize=on  Source_Type=DC  Amplitude=500  Phase=0  Frequency=0  Measurements=None
  Permanent Magnet Synchronous Machine : powerlib/Machines/Permanent Magnet Synchronous Machine  NbPhases=3  FluxDistribution=Trapezoidal  RotorType=Round  MechanicalLoad=Torque Tm  PresetModel=No  ShowDetailedParameters=on  MeasurementBus=off  Resistance=0.18  Inductance=0.000835  dqInductances=[8.5e-3, 8.5e-3]  La=0.000835  MachineConstant=Flux linkage established by magnets (V.s)  Flux=0.0142879  VoltageCst=44.8868  TorqueCst=0.42864  Flat=120  Mechanical=[0.00621417 0.000303448 15]  PolePairs=15  InitialConditions=[0,0, 0,0]  InitialConditions5ph=[0 0 0 0 0 0]  TsPowergui=0  TsBlock=-1  RefAngle=Aligned with phase A axis (original Park)
      settings: SourceProductName=Simscape Power Systems
  Universal Bridge1 : powerlib/Power Electronics/Universal Bridge  Arms=3  SnubberResistance=5000  SnubberCapacitance=inf  Device=MOSFET / Diodes  Ron=1e-3  Lon=0  ForwardVoltages="[  0  0  ]"  ForwardVoltage=0  GTOparameters=[ 10e-6 , 20e-6 ]  IGBTparameters=[ 1e-6 , 2e-6 ]  Measurements=None  Measurements_2=None  converterType=Rectifier
  Vab : Scope
  Vdc : Scope
  Voltage Measurement : powerlib/Measurements/Voltage Measurement  PhasorSimulation=off  OutputType=Complex  PSBequivalent=0
  Voltage Measurement1 : powerlib/Measurements/Voltage Measurement  PhasorSimulation=off  OutputType=Complex  PSBequivalent=0
  powergui : powerlib/powergui  Priority=2  SimulationMode=Discrete  SampleTime=Ts  frequency=60  Iterations=50  frequencyindice=0  Pbase=100e6  ErrMax=1e-4  UnitsV=kV  UnitsW=MW  buscounter=0  FunctionMessages=off  echomessages=off  EnableUseOfTLC=off  CurrentSourceSwitches=off  DisableSnubberDevices=off  DisableRonSwitches=off  DisableVfSwitches=off  DisplayEquations=off  SolverType=Tustin/Backward Euler (TBE)  Interpol=off  ExternalGateDelay=off  methode=off  Ts=0  x0status=blocks  SPID=off  SwTol=0  HookPort=off  RestoreLinks=warning  ResistiveCurrentMeasurement=off  Frange=[0:2:500]  Ylog=off  Xlog=on  ShowGrid=off  save=off  variable=ZData  structure=0  ZoomFFT=on  StartTime=0.0  cycles=1  DisplayStyle=1  fundamental=60  FreqAxis=off  MaxFrequency=1000  frequencyindicesteady=1  RmsSteady=1  display=off
  motor_out : Outport
  wires:
  Constant1/1 -> Controlled Voltage Source1/1
  Tm_Nm/1 -> Permanent Magnet Synchronous Machine/1
  gates_PWM/1 -> Universal Bridge1/1
  Voltage Measurement1/1 -> Vdc/1
  Permanent Magnet Synchronous Machine/1 -> motor_out/1
  Voltage Measurement/1 -> Vab/1
  connections:
  Voltage Measurement/LConn2 -- Permanent Magnet Synchronous Machine/LConn2 -- Universal Bridge1/LConn2
  Voltage Measurement1/LConn1 -- Controlled Voltage Source1/RConn1 -- Universal Bridge1/RConn1
  Universal Bridge1/RConn2 -- Controlled Voltage Source1/LConn1 -- Voltage Measurement1/LConn2
  Universal Bridge1/LConn3 -- Permanent Magnet Synchronous Machine/LConn3
  Universal Bridge1/LConn1 -- Permanent Magnet Synchronous Machine/LConn1 -- Voltage Measurement/LConn1

== system BLDCmotorControl_FOC_R2017b_fixdt/PWM_gates ==
  DC_pha : Inport
  Abs : Abs  OutDataTypeStr=Inherit: Inherit via back propagation  RndMeth=Zero
  Abs1 : Abs  OutDataTypeStr=Inherit: Inherit via back propagation  RndMeth=Zero
  Abs2 : Abs  OutDataTypeStr=Inherit: Inherit via back propagation  RndMeth=Zero
  Constant4 : Constant  Value=0  OutDataTypeStr=Inherit: Inherit via back propagation
  Demux : Demux  Outputs=3
  Gain8 : Gain  Gain=1/1000  OutDataTypeStr=Inherit: Inherit via back propagation  RndMeth=Zero
  MinMax : MinMax  Inputs=2  OutDataTypeStr=Inherit: Inherit via back propagation  RndMeth=Zero
  MinMax1 : MinMax  Function=max  Inputs=2  OutDataTypeStr=Inherit: Inherit via back propagation  RndMeth=Zero
  MinMax2 : MinMax  Inputs=2  OutDataTypeStr=Inherit: Inherit via back propagation  RndMeth=Zero
  MinMax3 : MinMax  Function=max  Inputs=2  OutDataTypeStr=Inherit: Inherit via back propagation  RndMeth=Zero
  MinMax4 : MinMax  Inputs=2  OutDataTypeStr=Inherit: Inherit via back propagation  RndMeth=Zero
  MinMax5 : MinMax  Function=max  Inputs=2  OutDataTypeStr=Inherit: Inherit via back propagation  RndMeth=Zero
  Mux4 : Mux  Inputs=6
  PWM_generator : pePwmGenerator/PWM Generator  Commented=on  CarrCount=Up  Tper=5e-5  Ts=5e-6
      settings: SourceProductName=The database C:\Users\37ef\AppData\Roaming\MathWorks\MATLAB\R2017b\slblocks_master.db is locked, or a table in the database is locked. (database is locked)
  PWM_generator1 : Subsystem
      mask help: Simulink:masks:GenSFuncDesc_MD
      mask Help: eval('feval(''rtwprivate'',''rtwhelpview'',''rtw_sfcn_block'')');
  PWM_generator12 : Subsystem
      mask help: Simulink:masks:GenSFuncDesc_MD
      mask Help: eval('feval(''rtwprivate'',''rtwhelpview'',''rtw_sfcn_block'')');
  PWM_generator2 : Subsystem
      mask help: Simulink:masks:GenSFuncDesc_MD
      mask Help: eval('feval(''rtwprivate'',''rtwhelpview'',''rtw_sfcn_block'')');
  PWM_generator3 : Subsystem
      mask help: Simulink:masks:GenSFuncDesc_MD
      mask Help: eval('feval(''rtwprivate'',''rtwhelpview'',''rtw_sfcn_block'')');
  PWM_generator4 : Subsystem
      mask help: Simulink:masks:GenSFuncDesc_MD
      mask Help: eval('feval(''rtwprivate'',''rtwhelpview'',''rtw_sfcn_block'')');
  PWM_generator5 : Subsystem
      mask help: Simulink:masks:GenSFuncDesc_MD
      mask Help: eval('feval(''rtwprivate'',''rtwhelpview'',''rtw_sfcn_block'')');
  signal_log6 : Subsystem
  gates_PWM : Outport
  wires:
  PWM_generator4/1(PWM) -> Mux4/5
  Abs/1 -> PWM_generator1/1(DC)
  PWM_generator12/1(PWM) -> Mux4/1
  PWM_generator5/1(PWM) -> Mux4/6
  MinMax1/1 -> PWM_generator12/1(DC)
  PWM_generator3/1(PWM) -> Mux4/4
  PWM_generator1/1(PWM) -> Mux4/2
  MinMax5/1 -> PWM_generator4/1(DC)
  PWM_generator2/1(PWM) -> Mux4/3
  Abs2/1 -> PWM_generator5/1(DC)
  MinMax3/1 -> PWM_generator2/1(DC)
  Abs1/1 -> PWM_generator3/1(DC)
  Demux/1 -> MinMax/2, MinMax1/2
  MinMax4/1 -> Abs2/1
  Constant4/1 -> MinMax1/1, MinMax4/1, MinMax5/1, MinMax2/1, MinMax3/1, MinMax/1
  MinMax2/1 -> Abs1/1
  Demux/2 -> MinMax2/2, MinMax3/2
  MinMax/1 -> Abs/1
  Demux/3 -> MinMax5/2, MinMax4/2
  DC_pha/1 -> Gain8/1
  Gain8/1 -> Demux/1
  Mux4/1 -> signal_log6/1(PWM), gates_PWM/1

== system BLDCmotorControl_FOC_R2017b_fixdt/Signal Builder ==
  Demux : Demux  Tag=STV Demux  Outputs=1
  FromWs : FromWorkspace  Tag=STV FromWs  VariableName=tuvar
      SigBuilderData=|
      | common.afterFinalStr = 'Extrapolate'
      | common.sampleTime = '-1'
      | dataSet.timeRange = [0 1.5]
      | dataSet.name = 'Group 1'
      | sbobj.Groups.Name = 'Group 1'
      | sbobj.Groups.Signals.Name = 'Signal 1'
      | sbobj.Groups.Signals.XData = [0 0.2 0.4 0.6 0.8 1.5]
      | sbobj.Groups.Signals.YData = [0 800 800 600 -800 -800]
      | sbobj.Groups.TimeRange = [0 1.5]
  Signal 1 : Outport  Tag=STV Outport
  wires:
  Demux/1 -> Signal 1/1
  FromWs/1 -> Demux/1

== system BLDCmotorControl_FOC_R2017b_fixdt/Theoretical_Speed_Trajectory ==
  note: Ideal Speed Trajectory Calculation
      | Based on Min/Max torque and Min/Max torque rate constraints
  r_inpTgtRaw : Inport
  Discrete Derivative1 : simulink/Discrete/Discrete Derivative  gainval=1.0  ICPrevScaledInput=0.0  OutMin=[]  OutMax=[]  OutDataType=fixdt(1, 16)  OutScaling=2^-10  DoSatur=off
  Discrete Derivative2 : simulink/Discrete/Discrete Derivative  gainval=1.0  ICPrevScaledInput=0.0  OutMin=[]  OutMax=[]  OutDataType=fixdt(1, 16)  OutScaling=2^-10  DoSatur=off
  Discrete-Time Integrator2 : DiscreteIntegrator  SampleTime=-1  ICPrevOutput=DiscIntNeverNeededParam  ICPrevScaledInput=DiscIntNeverNeededParam
  Divide2 : Product  Inputs=*/
  Divide3 : Product  Inputs=**
  Divide4 : Product  Inputs=**
  Gain1 : Gain  Gain=-1
  Gain2 : Gain  Gain=-1
  Gain4 : Gain  Gain=pi/30
  Gain5 : Gain  Gain=30/pi
  J_mot : Constant  Value=0.01  OutDataTypeStr=Inherit: Inherit via back propagation
  Kp : Constant  Value=65  OutDataTypeStr=Inherit: Inherit via back propagation
  M_max : Constant  Value=15  OutDataTypeStr=Inherit: Inherit via back propagation
  Manual Switch : ManualSwitch
  Mux4 : Mux  Inputs=2
  Rate Limiter Dynamic3 : simulink/Discontinuities/Rate Limiter Dynamic
      settings: SourceProductName=Simulink
  Saturation Dynamic : simulink/Discontinuities/Saturation Dynamic  OutMin=[]  OutMax=[]  OutDataTypeStr=Inherit: Same as second input  OutDataType=fixdt(1, 16)  OutScaling=2^-10  DoSatur=off
  Scope : Scope  NumInputPorts=3
  Sum2 : Sum  Inputs=|+-  RndMeth=Zero  OutDataTypeStr=Inherit: Same as first input
  Sum8 : Sum  Inputs=++|  RndMeth=Zero  OutDataTypeStr=Inherit: Same as first input
  dM_max : Constant  Value=500  OutDataTypeStr=Inherit: Inherit via back propagation
  r_inpTgt : Outport
  wires:
  Gain4/1 -> Divide4/2  "dw"
  M_max/1 -> Gain1/1, Saturation Dynamic/1
  J_mot/1 -> Divide2/2, Divide4/1
  Divide2/1 -> Gain5/1  "w"
  [r_inpTgtRaw] -> Discrete Derivative2/1, Sum2/1
  Divide4/1 -> Saturation Dynamic/2  "M"
  Gain1/1 -> Saturation Dynamic/3
  dM_max/1 -> Gain2/1, Rate Limiter Dynamic3/1
  Sum2/1 -> Divide3/2
  Divide3/1 -> Sum8/2
  Rate Limiter Dynamic3/1 -> [M_tgtTheo], Discrete-Time Integrator2/1
  Gain2/1 -> Rate Limiter Dynamic3/3
  Sum8/1 -> Gain4/1  "dn"
  Saturation Dynamic/1 -> Rate Limiter Dynamic3/2
  Gain5/1 -> [r_inpTgt], Sum2/2  "rpm"
  Kp/1 -> Divide3/1
  Discrete-Time Integrator2/1 -> Divide2/1
  Mux4/1 -> Scope/1
  Discrete Derivative1/1 -> Scope/3
  Discrete Derivative2/1 -> Sum8/1
  [M_tgtTheo] -> Discrete Derivative1/1, Scope/2
  r_inpTgtRaw/1 -> [r_inpTgtRaw]
  [r_inpTgtRaw] -> Mux4/1
  [r_inpTgt] -> Mux4/2
  [r_inpTgt] -> Manual Switch/2
  Manual Switch/1 -> r_inpTgt/1
  [r_inpTgtRaw] -> Manual Switch/1

== system BLDCmotorControl_FOC_R2017b_fixdt/filtLowPass ==
  u : Inport
  coef : Inport  Port=2
  Data Type Conversion : DataTypeConversion  OutDataTypeStr=fixdt(1,32,4)
  Low_Pass_Filter : Subsystem
      settings: RTWFcnNameOpts=Use subsystem name
      mask Display:
      | plot(0,0,100,100, ...
      | [73,75,73,75,25,25,28,25,22,25],[18,20,22,20,20,84,82,84,82,84], ...
      | [25,33,33,72],[20,20,70,70],[33,34,36,39,44,50,56,66,73],[20,25,33,43,55,63,66,70,70]);
      | text(50,40,'coef'),
  y : Outport
  wires:
  coef/1 -> Low_Pass_Filter/2(coef)
  u/1 -> Data Type Conversion/1
  Low_Pass_Filter/1(y) -> y/1
  Data Type Conversion/1 -> Low_Pass_Filter/1(u)

== system BLDCmotorControl_FOC_R2017b_fixdt/kph2rpm2 ==
  rad : Inport
  Constant : Constant  Value=360
  Constant1 : Constant  Value=n_polePairs
  Divide : Product  Inputs=**
  Gain4 : Gain  Gain=180/pi  RndMeth=Zero  OutDataTypeStr=Inherit: Same as input
  Math Function : Math  Operator=mod  SaturateOnIntegerOverflow=on
  deg : Outport
  wires:
  Math Function/1 -> deg/1
  rad/1 -> Gain4/1
  Constant/1 -> Math Function/2
  Gain4/1 -> Divide/1  "radps"
  Constant1/1 -> Divide/2
  Divide/1 -> Math Function/1

== system BLDCmotorControl_FOC_R2017b_fixdt/mixer ==
  speed : Inport
  steer : Inport  Port=2
  speed_coef : Inport  Port=3
  steer_coef : Inport  Port=4
  Data Type Conversion2 : DataTypeConversion  OutDataTypeStr=int16
  Data Type Conversion3 : DataTypeConversion  OutDataTypeStr=int16
  Data Type Conversion4 : DataTypeConversion  OutDataTypeStr=int16
  Display : Display
  Display1 : Display
  Display3 : Display
  Divide1 : Product  Inputs=**  RndMeth=Simplest  OutDataTypeStr=Inherit: Same as first input
  Divide2 : Product  Inputs=**  RndMeth=Simplest  OutDataTypeStr=Inherit: Same as first input
  Sum1 : Sum  Inputs=+-  RndMeth=Simplest  SaturateOnIntegerOverflow=on  InputSameDT=on  OutDataTypeStr=Inherit: Same as first input
  Sum2 : Sum  RndMeth=Simplest  SaturateOnIntegerOverflow=on  InputSameDT=on  OutDataTypeStr=Inherit: Same as first input
  speedR : Outport
  speedL : Outport  Port=2
  wires:
  Sum1/1 -> Data Type Conversion2/1
  speed/1 -> [speed]
  steer/1 -> [steer]
  speed_coef/1 -> [speed_coef]
  steer_coef/1 -> [steer_coef]
  [speed] -> Divide1/1
  [speed_coef] -> Divide1/2
  [steer] -> Divide2/1
  [steer_coef] -> Divide2/2
  Divide1/1 -> Display1/1, Data Type Conversion4/1, Sum2/1, Sum1/1
  Divide2/1 -> Sum2/2, Sum1/2
  Data Type Conversion2/1 -> speedR/1
  Data Type Conversion3/1 -> speedL/1
  Data Type Conversion4/1 -> Display/1
  Sum2/1 -> Display3/1, Data Type Conversion3/1

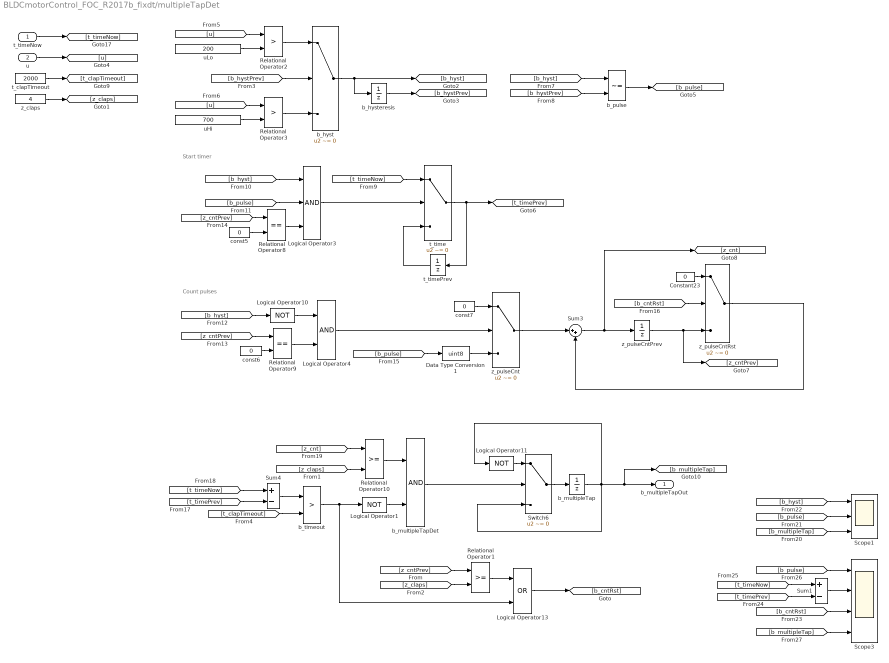
== system BLDCmotorControl_FOC_R2017b_fixdt/multipleTapDet ==
  note: Count pulses
  note: Start timer
  t_timeNow : Inport
  u : Inport  Port=2
  Constant23 : Constant  Value=0  OutDataTypeStr=Inherit: Inherit via back propagation
  Data Type Conversion1 : DataTypeConversion  OutDataTypeStr=uint8
  Logical Operator1 : Logic  Operator=NOT  AllPortsSameDT=off  OutDataTypeStr=boolean
  Logical Operator10 : Logic  Operator=NOT  AllPortsSameDT=off  OutDataTypeStr=boolean
  Logical Operator11 : Logic  Operator=NOT  AllPortsSameDT=off  OutDataTypeStr=boolean
  Logical Operator13 : Logic  Operator=OR  AllPortsSameDT=off  OutDataTypeStr=boolean
  Logical Operator3 : Logic  Inputs=3  AllPortsSameDT=off  OutDataTypeStr=boolean
  Logical Operator4 : Logic  AllPortsSameDT=off  OutDataTypeStr=boolean
  Relational Operator1 : RelationalOperator  OutDataTypeStr=boolean  RndMeth=Simplest
  Relational Operator10 : RelationalOperator  OutDataTypeStr=boolean  RndMeth=Simplest
  Relational Operator2 : RelationalOperator  Operator=>  OutDataTypeStr=boolean  RndMeth=Simplest
  Relational Operator3 : RelationalOperator  Operator=>  OutDataTypeStr=boolean  RndMeth=Simplest
  Relational Operator8 : RelationalOperator  Operator===  OutDataTypeStr=boolean  RndMeth=Simplest
  Relational Operator9 : RelationalOperator  Operator===  OutDataTypeStr=boolean  RndMeth=Simplest
  Scope1 : Scope  NumInputPorts=3
  Scope3 : Scope  NumInputPorts=4
  Sum1 : Sum  Inputs=+-
  Sum3 : Sum  Inputs=|++
  Sum4 : Sum  Inputs=+-
  Switch6 : Switch  Criteria=u2 ~= 0  OutDataTypeStr=Inherit: Inherit via back propagation  RndMeth=Zero
  b_hyst : Switch  Criteria=u2 ~= 0  RndMeth=Zero
  b_hysteresis : UnitDelay  SampleTime=-1
      settings: AttributesFormatString=Ini=%<X0>
  b_multipleTap : UnitDelay  SampleTime=-1
      settings: AttributesFormatString=Ini=%<X0>
  b_multipleTapDet : Logic  AllPortsSameDT=off  OutDataTypeStr=boolean
  b_pulse : RelationalOperator  Operator=~=  OutDataTypeStr=boolean  RndMeth=Simplest
  b_timeout : RelationalOperator  Operator=>  OutDataTypeStr=boolean  RndMeth=Simplest
  const5 : Constant  Value=0  OutDataTypeStr=Inherit: Inherit via back propagation
  const6 : Constant  Value=0  OutDataTypeStr=Inherit: Inherit via back propagation
  const7 : Constant  Value=0  OutDataTypeStr=Inherit: Inherit via back propagation
  t_clapTimeout : Constant  Value=2000  OutDataTypeStr=Inherit: Inherit via back propagation
  t_time : Switch  Criteria=u2 ~= 0  OutDataTypeStr=Inherit: Inherit via back propagation  RndMeth=Zero
  t_timePrev : UnitDelay  SampleTime=-1
      settings: AttributesFormatString=Ini=%<X0>
  uHi : Constant  Value=700  OutDataTypeStr=Inherit: Inherit via back propagation
  uLo : Constant  Value=200  OutDataTypeStr=Inherit: Inherit via back propagation
  z_claps : Constant  Value=4  OutDataTypeStr=Inherit: Inherit via back propagation
  z_pulseCnt : Switch  Criteria=u2 ~= 0  OutDataTypeStr=Inherit: Inherit via back propagation  RndMeth=Zero
  z_pulseCntPrev : UnitDelay  SampleTime=-1
      settings: AttributesFormatString=Ini=%<X0>
  z_pulseCntRst : Switch  Criteria=u2 ~= 0  OutDataTypeStr=Inherit: Inherit via back propagation  RndMeth=Simplest
  b_multipleTapOut : Outport
  wires:
  t_timeNow/1 -> [t_timeNow]
  Relational Operator2/1 -> b_hyst/1
  b_hyst/1 -> b_hysteresis/1, [b_hyst]
  uLo/1 -> Relational Operator2/2
  b_hysteresis/1 -> [b_hystPrev]
  [b_hystPrev] -> b_hyst/2
  uHi/1 -> Relational Operator3/2
  Relational Operator3/1 -> b_hyst/3
  u/1 -> [u]
  [u] -> Relational Operator2/1
  [u] -> Relational Operator3/1
  [b_hyst] -> b_pulse/1
  [b_hystPrev] -> b_pulse/2
  b_pulse/1 -> [b_pulse]
  t_time/1 -> t_timePrev/1, [t_timePrev]
  t_timePrev/1 -> t_time/3
  [t_timeNow] -> t_time/1
  const5/1 -> Relational Operator8/2
  Relational Operator8/1 -> Logical Operator3/3
  Logical Operator3/1 -> t_time/2
  [b_hyst] -> Logical Operator3/1
  [b_pulse] -> Logical Operator3/2
  Data Type Conversion1/1 -> z_pulseCnt/3
  const7/1 -> z_pulseCnt/1
  Logical Operator4/1 -> z_pulseCnt/2
  const6/1 -> Relational Operator9/2
  Relational Operator9/1 -> Logical Operator4/2
  Logical Operator10/1 -> Logical Operator4/1
  [b_pulse] -> Data Type Conversion1/1
  [b_hyst] -> Logical Operator10/1
  [z_cntPrev] -> Relational Operator9/1
  [z_cntPrev] -> Relational Operator8/1
  z_pulseCnt/1 -> Sum3/1
  Sum4/1 -> b_timeout/1
  [t_timePrev] -> Sum4/2
  [t_timeNow] -> Sum4/1
  [t_clapTimeout] -> b_timeout/2
  Logical Operator11/1 -> Switch6/1
  b_multipleTap/1 -> Switch6/3, [b_multipleTap], b_multipleTapOut/1, Logical Operator11/1
  Switch6/1 -> b_multipleTap/1
  [z_claps] -> Relational Operator10/2
  [z_cnt] -> Relational Operator10/1
  Relational Operator10/1 -> b_multipleTapDet/1
  b_timeout/1 -> Logical Operator13/2, Logical Operator1/1
  [b_pulse] -> Scope1/2
  [b_hyst] -> Scope1/1
  b_multipleTapDet/1 -> Switch6/2
  Logical Operator13/1 -> [b_cntRst]
  [z_cntPrev] -> Relational Operator1/1
  [z_claps] -> Relational Operator1/2
  Relational Operator1/1 -> Logical Operator13/1
  [b_cntRst] -> z_pulseCntRst/2
  Constant23/1 -> z_pulseCntRst/1
  z_pulseCntPrev/1 -> [z_cntPrev], z_pulseCntRst/3
  z_pulseCntRst/1 -> Sum3/2
  z_claps/1 -> [z_claps]
  t_clapTimeout/1 -> [t_clapTimeout]
  Logical Operator1/1 -> b_multipleTapDet/2
  Sum3/1 -> [z_cnt], z_pulseCntPrev/1
  [t_timeNow] -> Sum1/1
  [t_timePrev] -> Sum1/2
  [b_pulse] -> Scope3/1
  Sum1/1 -> Scope3/2
  [b_cntRst] -> Scope3/3
  [b_multipleTap] -> Scope1/3
  [b_multipleTap] -> Scope3/4
